simulink model "sample_model"  (R2016b)
settings: Solver=FixedStepDiscrete  StartTime=0.0  StopTime=10  RelTol=1e-3
settings Model: Creator=40005102  LastModifiedBy=40005102

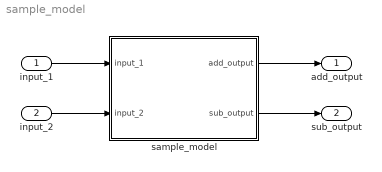
== system sample_model ==
  input_1 : Inport
  input_2 : Inport  Port=2
  sample_model : Subsystem
  add_output : Outport
  sub_output : Outport  Port=2
  wires:
  input_1/1 -> sample_model/1(input_1)
  input_2/1 -> sample_model/2(input_2)
  sample_model/1(add_output) -> add_output/1
  sample_model/2(sub_output) -> sub_output/1

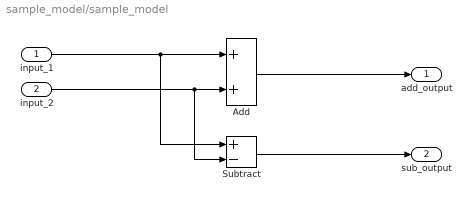
== system sample_model/sample_model ==
  input_1 : Inport
  input_2 : Inport  Port=2
  Add : Sum
  Subtract : Sum  Inputs=+-
  add_output : Outport
  sub_output : Outport  Port=2
  wires:
  input_2/1 -> Subtract/2, Add/2
  Add/1 -> add_output/1
  Subtract/1 -> sub_output/1
  input_1/1 -> Subtract/1, Add/1
